simulink model "rover_control"  (R2019b)
settings: Solver=ode3  StartTime=0.0  StopTime=inf  RelTol=1e-3  EnableMultiTasking=on
undefined symbols (not defined in the file or in its folder): Discrete, Time
libraries: embdlinuxlib x13, simulink x3, ctrlSharedLib x2, raspberrypilib x2, sensehatlib x1
(part 1 of 2)
settings Model: DataDictionary=common.sldd  FPTRunName=Active  SimulationMode=external  ExtModeBatchMode=on  ExtModeTrigDuration=100  ExtModeArchiveFileName=rover  ExtModeArchiveDirName=C:\Users\nmb\Desktop\MarsRover\log  ExtModeAddSuffixToVar=on  Creator=nmb  LastModifiedBy=nmb
settings SolverCC: PositivePriorityOrder=on
settings DataIOCC: LimitDataPoints=on  SaveFormat=Array
settings OptimizationCC: ExpressionDepthLimit=2147483647  LifeSpan=Inf  MaxStackSize=64
settings DebuggingCC: UnderspecifiedInitializationDetection=Classic  MergeDetectMultiDrivingBlocksExec=none  FcnCallInpInsideContextMsg=warning  AllowSymbolicDim=off  StateNameClashWarn=warning  SFUnexpectedBacktrackingDiag=warning  SFNoUnconditionalDefaultTransitionDiag=warning  SFExecutionAtInitializationDiag=none  ArithmeticOperatorsInVariantConditions=warning
settings HardwareCC: ProdBitPerPointer=32  ProdBitPerSizeT=32  ProdBitPerPtrDiffT=32  ProdLargestAtomicInteger=Long  ProdLargestAtomicFloat=Double  ProdWordSize=32  ProdHWDeviceType=ARM Compatible->ARM Cortex  UseEmbeddedCoderFeatures=off
settings ModelReferenceCC: PropagateSignalLabelsOutOfModel=off
settings SFSimCC: SimUseLocalCustomCode=off  CustomCodeUndefinedFunction=UseInterfaceOnly
settings RTWCC: SystemTargetFile=ert.tlc  HardwareBoard=Raspberry Pi  TemplateMakefile=ert_default_tmf  GenerateReport=on  RTWVerbose=off  RTWUseLocalCustomCode=off  Toolchain=GNU GCC Raspberry Pi  BuildConfiguration=Faster Runs  LaunchReport=on
settings CodeAppCC: ForceParamTrailComments=on  OperatorAnnotations=on  StateflowObjectComments=on  MATLABSourceComments=on
settings ERTTargetCC: MultiwordLength=2048  ERTCustomFileBanners=off  SupportContinuousTime=on  SupportNonInlinedSFcns=on  RemoveResetFunc=off  SupportVariableSizeSignals=on  ModelStepFunctionPrototypeControlCompliant=off  ExtMode=on  ExtModeMexArgs='192.168.35.184' 0 17725  ERTSrcFileBannerTemplate=codertarget_code_template.cgt  ERTHdrFileBannerTemplate=codertarget_code_template.cgt  ERTDataSrcFileTemplate=codertarget_code_template.cgt  ERTDataHdrFileTemplate=codertarget_code_template.cgt
settings ConfigComp: CovMetricSettings=dw  CovHtmlReporting=on  CovSaveCumulativeToWorkspaceVar=on  CovSaveSingleToWorkspaceVar=on  CovExternalEMLEnable=off  CovSFcnEnable=off

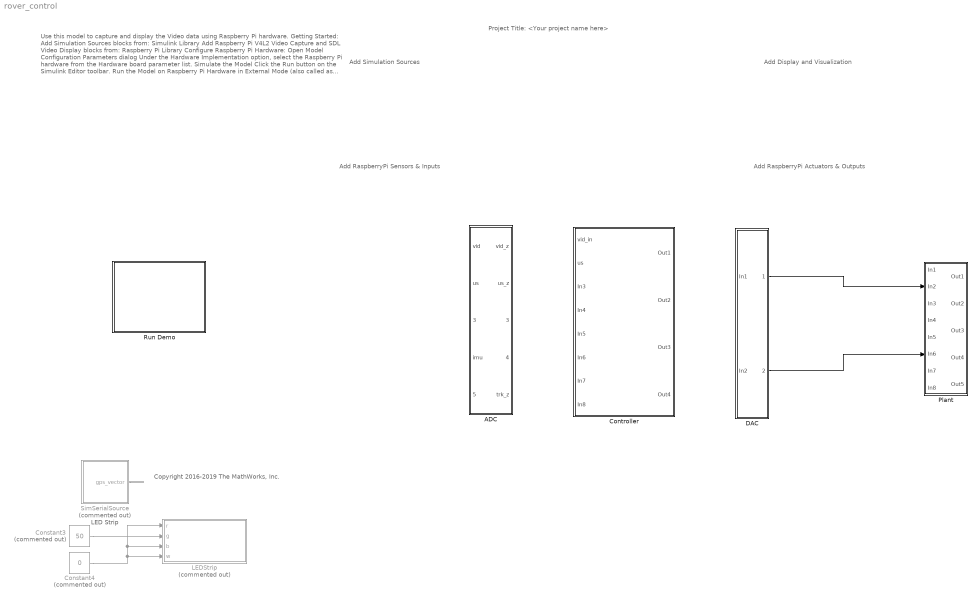
== system rover_control ==
  note: LED Strip
  note: Use this model to capture and display the Video data using Raspberry Pi hardware.
      |
      | Getting Started:
      |
      | Add Simulation Sources blocks from:
      | Simulink Library
      | Add Raspberry Pi V4L2 Video Capture and SDL Video Display blocks from:
      | Raspberry Pi Library
      |
      | Configure Raspberry Pi Hardware:
      |
      | Open Model Configuration Parameters dialog
      | Under the Hardware Implementation option, select the Raspberry Pi hardware from the Hardware board parameter list.
      |
      | Simulate the Model
      |
      | Click the Run button on the Simulink Editor toolbar.
      |
      | Run the Model on Raspberry Pi Hardware in External Mode (also called as Monitor & Tune)
      |
      | In the Hardware tab, click Monitor & Tune
      |
      | External mode will stop when the number of seconds specified in the Simulation stop time parameter elapses.
      |
      | Learn More
      |
      | V4L2 Video Capture
      |
      | SDL Video Display
  note: Add RaspberryPi Sensors & Inputs
  note: Add Display and Visualization
  note: Project Title: <Your project name here>
  note: Add RaspberryPi Actuators & Outputs
  note: Add Simulation Sources
  note: Copyright 2016-2019 The MathWorks, Inc.
  ADC : Subsystem
  Constant3 : Constant  Commented=on  Value=50  OutDataTypeStr=Inherit: Inherit via back propagation
  Constant4 : Constant  Commented=on  Value=0  OutDataTypeStr=Inherit: Inherit via back propagation
  Controller : Subsystem
  DAC : Subsystem
  LEDStrip : Subsystem  Commented=on  DialogController=linuxDDGCreate  InitFcn=|  mask(Ultrasonic Read){board=Model B+, gpio=12, internalResistor=Off, sampleTime=1, direction=Input, blockPlatform=Raspberry Pi}
      | realtime.internal.validateLinuxBlock(get_param(gcbh,'blockPlatform'), gcbh);
      | realtime.internal.gpioCheckParameters(gcs,gcb);
      | realtime.internal.validateGPIO(gcb);
      mask prompts: gpio "GPIO number:"; internalResistor "Internal resistor:"; sampleTime "Sample time:"; blockPlatform "Block platform:"
      mask help: Reads the logical value of a specified GPIO pin configured as input. Select the GPIO input number. Select the internal resistor. Use only one block per GPIO.
      mask init:
      | h = realtime.internal.BoardInfo(blockPlatform);
      | gpioPinName = h.getGPIOPrimaryFunction(board, gpio);
      | gpioPinName = uint8([gpioPinName, 0]); % Add C string termination character
      | 
      | switch (internalResistor)
      |     case {'Off'}
      |         resistor = 1;
      |     case {'Pull-up'}
      |         resistor = 2;
      |     case {'Pull-down'}
      |         resistor = 3;
      |     otherwise
      |         resistor = 255; %N/A
      | end
      | realtime.internal.linuxGpioRead('MaskInitialization');
      mask Help: eval('realtime.helpView(get_param(gcb, ''blockPlatform''), [realtime.internal.getHelpLinkPrefix(gcb) ''libgpioread''])');
      mask TypeOptions direction: Input | Output
      mask Display:
      | text(0.5, 0.15, 'GPIO 12', 'horizontalAlignment', 'center');
      | image(imread('digitalio.png'),[0.32 0.25 0.35 0.55]);
      | color('blue');
      | text(0.90, 0.90, 'RASPBERRYPI', 'horizontalAlignment', 'right');
      | color('black');
  Plant : Subsystem
  Run Demo : Subsystem  Description=Controls host-side RTDX processing.
      mask Display: pic=imread('raspberrypiMonitorAndTune.png');image(pic);
  SimSerialSource : Subsystem  Commented=on
  wires:
  Constant3/1 -> LEDStrip/2(g)
  Constant4/1 -> LEDStrip/1(r), LEDStrip/3(b), LEDStrip/4(w)
  SimSerialSource/1(gps_vector) -> ?
  ? -> ADC/1(vid)
  ? -> ADC/2(us)
  ? -> ADC/3(gps_ser)
  ? -> ADC/4(imu)
  ? -> ADC/5(tracking)
  DAC/1(Out1) -> Plant/2(In2)
  DAC/2(Out2) -> Plant/6(In6)

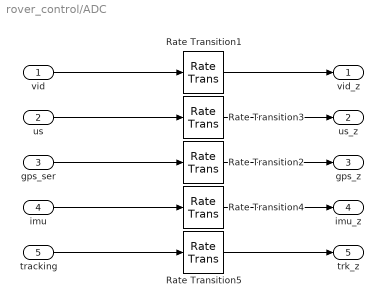
== system rover_control/ADC ==
  vid : Inport
  us : Inport  Port=2
  gps_ser : Inport  Port=3
  imu : Inport  Port=4
  tracking : Inport  Port=5
  Rate Transition{1..5} (5 alike) : RateTransition
  vid_z : Outport
  us_z : Outport  Port=2
  gps_z : Outport  Port=3
  imu_z : Outport  Port=4
  trk_z : Outport  Port=5
  wires:
  Rate Transition3/1 -> us_z/1
  us/1 -> Rate Transition3/1
  vid/1 -> Rate Transition1/1
  Rate Transition1/1 -> vid_z/1
  Rate Transition2/1 -> gps_z/1
  Rate Transition4/1 -> imu_z/1
  gps_ser/1 -> Rate Transition2/1
  imu/1 -> Rate Transition4/1
  tracking/1 -> Rate Transition5/1
  Rate Transition5/1 -> trk_z/1

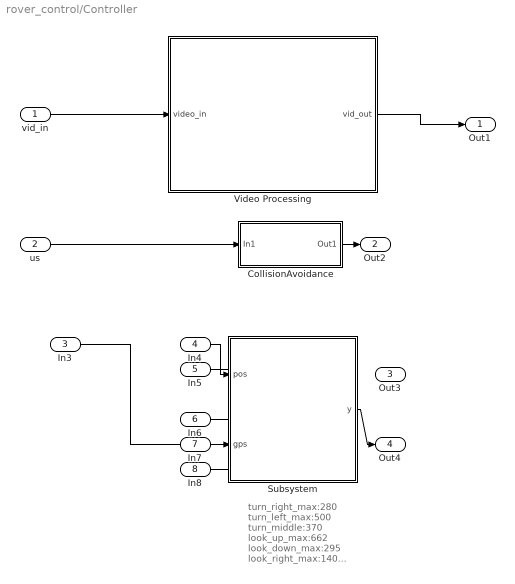
== system rover_control/Controller ==
  note: turn_right_max:280
      | turn_left_max:500
      | turn_middle:370
      | look_up_max:662
      | look_down_max:295
      | look_right_max:140
      | look_left_max:476
  vid_in : Inport
  us : Inport  Port=2
  In3 : Inport  Port=3
  In4 : Inport  Port=4
  In5 : Inport  Port=5
  In6 : Inport  Port=6
  In7 : Inport  Port=7
  In8 : Inport  Port=8
  CollisionAvoidance : Subsystem
  Subsystem : Subsystem
  Video Processing : Subsystem
  Out1 : Outport
  Out2 : Outport  Port=2
  Out3 : Outport  Port=3
  Out4 : Outport  Port=4
  wires:
  In8/1 -> ?
  ? -> Out3/1
  In5/1 -> ?
  vid_in/1 -> Video Processing/1(video_in)
  In7/1 -> ?
  CollisionAvoidance/1(Out1) -> Out2/1
  us/1 -> CollisionAvoidance/1(In1)
  In4/1 -> Subsystem/1(pos)
  In6/1 -> ?
  Subsystem/1(y) -> Out4/1
  In3/1 -> Subsystem/2(gps)
  Video Processing/1(vid_out) -> Out1/1

== system rover_control/DAC ==
  In1 : Inport
  In2 : Inport  Port=2
  Rate Transition : RateTransition  OutPortSampleTime=0.5
  Rate Transition1 : RateTransition  OutPortSampleTime=0.5
  Out1 : Outport
  Out2 : Outport  Port=2
  wires:
  In2/1 -> Rate Transition1/1
  In1/1 -> Rate Transition/1
  Rate Transition1/1 -> Out2/1
  Rate Transition/1 -> Out1/1

== system rover_control/LEDStrip ==
  r : Inport
  g : Inport  Port=2
  b : Inport  Port=3
  w : Inport  Port=4
  MATLAB System : MATLABSystem  System=WS2812  OutputPin=gpio  SampleTime=sampleTime
      mask Type: WS2812
      mask Display: disp('WS2812');
  wires:
  r/1 -> MATLAB System/1
  g/1 -> MATLAB System/2
  b/1 -> MATLAB System/3
  w/1 -> MATLAB System/4

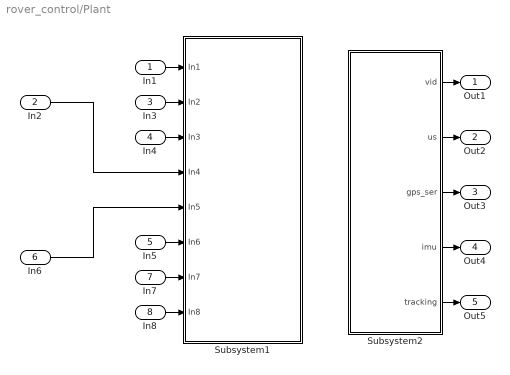
== system rover_control/Plant ==
  In1 : Inport
  In2 : Inport  Port=2
  In3 : Inport  Port=3
  In4 : Inport  Port=4
  In5 : Inport  Port=5
  In6 : Inport  Port=6
  In7 : Inport  Port=7
  In8 : Inport  Port=8
  Subsystem1 : Subsystem  VariantControlMode=Label  Variant=on  VariantControl=Variant1  LabelModeActiveChoice=Variant1
  Subsystem2 : Subsystem  VariantControlMode=Label  Variant=on  VariantControl=Variant1  LabelModeActiveChoice=Variant1
  Out1 : Outport
  Out2 : Outport  Port=2
  Out3 : Outport  Port=3
  Out4 : Outport  Port=4
  Out5 : Outport  Port=5
  wires:
  In3/1 -> Subsystem1/2(In2)
  Subsystem2/2(us) -> Out2/1
  Subsystem2/3(gps_ser) -> Out3/1
  Subsystem2/4(imu) -> Out4/1
  Subsystem2/1(vid) -> Out1/1
  In8/1 -> Subsystem1/8(In8)
  Subsystem2/5(tracking) -> Out5/1
  In2/1 -> Subsystem1/4(In4)
  In7/1 -> Subsystem1/7(In7)
  In6/1 -> Subsystem1/5(In5)
  In1/1 -> Subsystem1/1(In1)
  In4/1 -> Subsystem1/3(In3)
  In5/1 -> Subsystem1/6(In6)

== system rover_control/Run Demo ==

== system rover_control/SimSerialSource ==
  Zero : Constant  Value=uint8(zeros(1,164))  OutDataTypeStr=Inherit: Inherit via back propagation
  gps_vector : Outport
  wires:
  Zero/1 -> gps_vector/1  "gps_vector"

== system rover_control/Controller/CollisionAvoidance ==
  In1 : Inport  SampleTime=0.06
  Chart : Stateflow chart  BlockKeywords=__PRM__SERIALIZED__DATA__:Stateflow Chart,Stateflow Diagram  TreatAsAtomicUnit=on
  Ground : Ground
  Kalman Filter : ctrlSharedLib/Kalman Filter  TimeDomain=Discrete-Time  UseCurrentEstimator=on  ModelSource=Individual A, B, C, D matrices  ModelSourceVariable=ss(0.95,1,1,0,1)  A=[1 0.06; 0 1]  B=1  C=[1 1]  D=0  NumberOfStates=1  NumberOfInputs=1  NumberOfOutputs=1  InitialEstimateSource=Dialog  X0=0  P0=10  UseK=off  UseGH=off  NumberOfProcessNoiseInputs=1  G=[0.1/2 0;1 0]  TimeInvariantG=on  H=0  TimeInvariantH=on  Q=0.05  TimeInvariantQ=on  R=50  TimeInvariantR=on  N=0  TimeInvariantN=on  AddInputPort=off  AddEnablePort=off  OutputEstimatedY=off  OutputP=off  Ts=0.06
      settings: SourceProductBaseCode=CT
  Scope : Scope  NumInputPorts=2
  Out1 : Outport
  wires:
  Kalman Filter/1 -> Scope/2, Chart/1(data)
  Ground/1 -> Out1/1
  In1/1 -> Scope/1, Kalman Filter/1

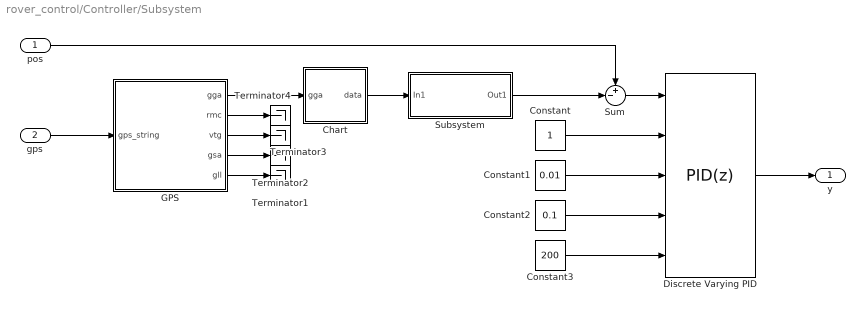
== system rover_control/Controller/Subsystem ==
  pos : Inport
  gps : Inport  Port=2
  Chart : Stateflow chart  BlockKeywords=__PRM__SERIALIZED__DATA__:Stateflow Chart,Stateflow Diagram  TreatAsAtomicUnit=on
  Constant : Constant
  Constant1 : Constant  Value=0.01
  Constant2 : Constant  Value=0.1
  Constant3 : Constant  Value=200
  Discrete Varying PID : simulink/Continuous/PID Controller  Controller=PID  Form=Parallel  TimeDomain=Discrete-time  SampleTime=-1  IntegratorMethod=Forward Euler  FilterMethod=Forward Euler  ControllerParametersSource=external  P=1  I=1  D=0  UseFilter=on  N=100  TunerSelectOption=Transfer Function Based (PID Tuner App)  InitialConditionSource=internal  InitialConditionForIntegrator=0  InitialConditionForFilter=0  DifferentiatorICPrevScaledInput=0  ExternalReset=none  TrackingMode=off  Kt=1  LimitOutput=off  UpperSaturationLimit=inf  LowerSaturationLimit=-inf  LinearizeAsGain=on  AntiWindupMode=none  Kb=1  POutMin=[]  POutMax=[]  IOutMin=[]  IOutMax=[]  DOutMin=[]  DOutMax=[]  NOutMin=[]  NOutMax=[]  SumOutMin=[]  SumOutMax=[]  SaturationOutMin=[]  SaturationOutMax=[]  PParamMin=[]  PParamMax=[]  IParamMin=[]  IParamMax=[]  DParamMin=[]  DParamMax=[]  NParamMin=[]  NParamMax=[]  KbParamMin=[]  KbParamMax=[]  KtParamMin=[]  KtParamMax=[]  KbOutMin=[]  KbOutMax=[]  KtOutMin=[]  KtOutMax=[]  IntegratorOutMin=[]  IntegratorOutMax=[]  FilterOutMin=[]  FilterOutMax=[]  SumI1OutMin=[]  SumI1OutMax=[]  SumI2OutMin=[]  SumI2OutMax=[]  SumI3OutMin=[]  SumI3OutMax=[]  SumI4OutMin=[]  SumI4OutMax=[]  SumDOutMin=[]  SumDOutMax=[]  DifferentiatorOutMin=[]  DifferentiatorOutMax=[]  FilterDiffOutCoefMin=[]  FilterDiffOutCoefMax=[]  ReciprocalOutMin=[]  ReciprocalOutMax=[]  SumDenOutMin=[]  SumDenOutMax=[]  SumNumOutMin=[]  SumNumOutMax=[]  DivideOutMin=[]  DivideOutMax=[]  IntegratorContinuousStateAttributes=''  IntegratorStateMustResolveToSignalObject=off  IntegratorRTWStateStorageClass=Auto  FilterContinuousStateAttributes=''  FilterStateMustResolveToSignalObject=off  FilterRTWStateStorageClass=Auto  ParallelPVariant=ExternalParameters  IdealPVariant=Disabled  IVariant=ExternalParameters  DVariant=ExternalParameters  IntegratorVariant=Discrete  SatVariant=Disabled  AWVariant=Passthrough  PCopyVariant=Disabled  TRVariant=Disabled  FdbkBlocksVariant=Forward  IdealPFdbkVariant=Disabled  SatFdbkVariant=Disabled  DerivativeFilterVariant=ForwardEulerFilter  NVariant=ExternalParameters  NCopyVariant=Disabled  FilterICVariant=InternalICsFilter  IntegratorICVariant=InternalICs  ExternalResetVariant=Disabled  TRSumVariant=Passthrough  SumFdbkVariant=Disabled  SumVariant=Sum_PID
  GPS : Subsystem
  Subsystem : Subsystem
  Sum : Sum  Inputs=+-|
  Terminator{1..4} (4 alike) : Terminator
  y : Outport
  wires:
  GPS/5(gll) -> Terminator1/1
  pos/1 -> Sum/1
  GPS/3(vtg) -> Terminator3/1
  GPS/4(gsa) -> Terminator2/1
  Constant3/1 -> Discrete Varying PID/5
  Constant/1 -> Discrete Varying PID/2
  Constant2/1 -> Discrete Varying PID/4
  GPS/2(rmc) -> Terminator4/1
  GPS/1(gga) -> Chart/1(gga)
  Discrete Varying PID/1 -> y/1
  Constant1/1 -> Discrete Varying PID/3
  gps/1 -> GPS/1(gps_string)
  Chart/1(data) -> Subsystem/1(In1)
  Sum/1 -> Discrete Varying PID/1
  Subsystem/1(Out1) -> Sum/2

== system rover_control/Controller/Video Processing ==
  video_in : Inport
  vid_out : Outport
  wires:
  video_in/1 -> vid_out/1

== system rover_control/Plant/Subsystem1 ==
  In1 : Inport
  In2 : Inport  Port=2
  In3 : Inport  Port=3
  In4 : Inport  Port=4
  In5 : Inport  Port=5
  In6 : Inport  Port=6
  In7 : Inport  Port=7
  In8 : Inport  Port=8
  Subsystem1 : Subsystem  VariantControl=Variant1

== system rover_control/Plant/Subsystem2 ==
  RPiSystem : Subsystem  VariantControl=Variant1
  vid : Outport
  us : Outport  Port=2
  gps_ser : Outport  Port=3
  imu : Outport  Port=4
  tracking : Outport  Port=5

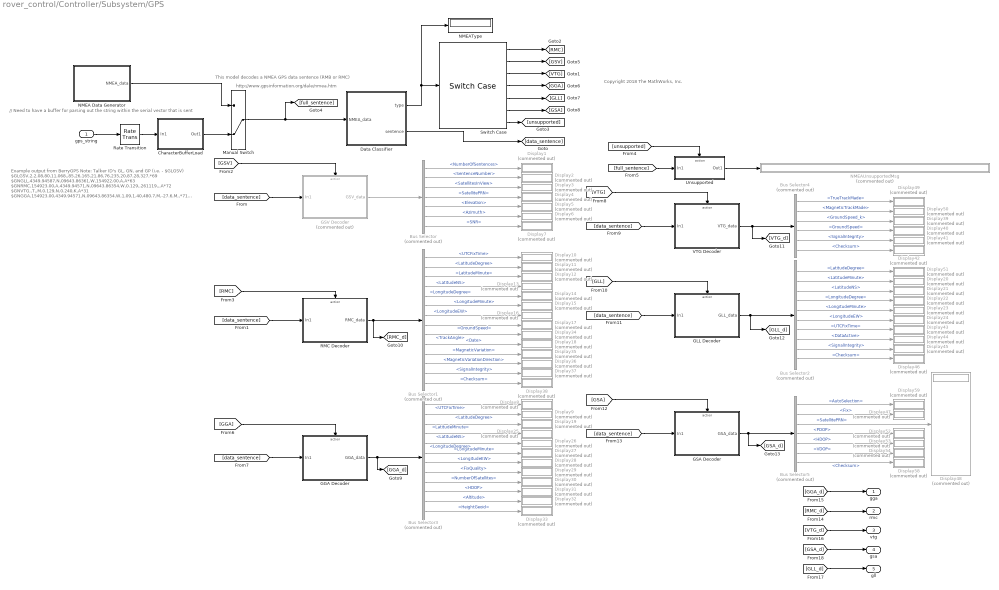
== system rover_control/Controller/Subsystem/GPS ==
  note: // Need to have a buffer for parsing out the string within the serial vector that is sent
  note: Example output from BerryGPS
      | Note: Talker ID's GL, GN, and GP (i.e. - $GLGSV)
      |
      | $GLGSV,2,2,08,80,11,068,,85,26,165,21,86,76,235,20,87,28,327,*69
      | $GNGLL,4349.94587,N,09643.86361,W,154922.00,A,A*63
      | $GNRMC,154923.00,A,4349.94571,N,09643.86354,W,0.129,,261119,,,A*72
      | $GNVTG,,T,,M,0.129,N,0.240,K,A*31
      | $GNGGA,154923.00,4349.94571,N,09643.86354,W,1,09,1.40,480.7,M,-27.6,M,,*71
      | $GNGSA,A,3,32,21,20,29,13,15,,,,,,,1.95,1.40,1.35*1E
      | $GNGSA,A,3,85,71,70,,,,,,,,,,1.95,1.40,1.35*1F
      | $GPGSV,3,1,10,08,05,331,,10,41,276,19,13,19,044,11,15,49,058,26*73
      | $GPGSV,3,2,10,20,68,302,16,21,84,181,17,24,25,126,15,27,28,306,*78
      | $GPGSV,3,3,10,29,09,180,12,32,10,214,27*72
      | $GLGSV,2,1,08,70,31,044,15,71,73,335,10,72,36,249,,79,08,018,*69
      | $GLGSV,2,2,08,80,11,068,,85,26,165,20,86,76,235,20,87,28,327,*68
      | $GNGLL,4349.94571,N,09643.86354,W,154923.00,A,A*6D
      | $GNRMC,154924.00,A,4349.94580,N,09643.86402,W,0.280,,261119,,,A*7F
      | $GNVTG,,T,,M,0.280,N,0.518,K,A*3B
      | $GNGGA,154924.00,4349.94580,N,09643.86402,W,1,09,1.40,481.1,M,-27.6,M,,*7B
      | $GNGSA,A,3,32,21,20,29,13,15,,,,,,,1.95,1.40,1.35*1E
      | $GNGSA,A,3,85,71,70,,,,,,,,,,1.95,1.40,1.35*1F
      | $GPGSV,3,1,10,08,05,331,,10,41,276,19,13,19,044,11,15,49,058,27*72
      | $GPGSV,3,2,10,20,68,303,17,21,84,181,18,24,25,126,15,27,28,306,*77
      | $GPGSV,3,3,10,29,09,180,10,32,10,214,27*70
      | $GLGSV,2,1,08,70,31,044,11,71,73,335,10,72,36,249,,79,08,018,*6D
      | $GLGSV,2,2,08,80,11,068,,85,26,165,21,86,76,235,20,87,28,327,*69
      | $GNGLL,4349.94580,N,09643.86402,W,154924.00,A,A*60
      | $GNRMC,154925.00,A,4349.94623,N,09643.86468,W,0.724,,261119,,,A*73
      | $GNVTG,,T,,M,0.724,N,1.340,K,A*3A
      | $GNGGA,154925.00,4349.94623,N,09643.86468,W,1,09,1.40,480.9,M,-27.6,M,,*75
      | $GNGSA,A,3,32,21,20,29,13,15,,,,,,,1.95,1.40,1.35*1E
      | $GNGSA,A,3,85,71,70,,,,,,,,,,1.95,1.40,1.35*1F
      | $GPGSV,3,1,10,08,05,331,,10,41,276,19,13,19,044,12,15,49,058,27*71
      | $GPGSV,3,2,10,20,68,303,16,21,84,179,18,24,25,126,13,27,28,306,*77
      | $GPGSV,3,3,10,29,09,180,13,32,10,214,27*73
      | $GLGSV,2,1,08,70,31,044,11,71,73,335,07,72,36,249,,79,08,018,*6B
      | $GLGSV,2,2,08,80,11,068,,85,26,165,21,86,76,235,20,87,28,327,*69
      | $GNGLL,4349.94623,N,09643.86468,W,154925.00,A,A*67
  note: Copyright 2018 The MathWorks, Inc.
  note: This model decodes a NMEA GPS data sentence (RMB or RMC)
  note: http://www.gpsinformation.org/dale/nmea.htm
  gps_string : Inport
  Bus Selector : BusSelector  Commented=on  OutputSignals=NumberOfSentences,SentenceNumber,SatellitesInView,SatellitePRN,Elevation,Azimuth,SNR
  Bus Selector1 : BusSelector  Commented=on  OutputSignals=UTCFixTime,LatitudeDegree,LatitudeMinute,LatitudeNS,LongitudeDegree,LongitudeMinute,LongitudeEW,GroundSpeed,TrackAngle,Date,MagneticVariation,MagneticVariationDirection,SignalIntegrity,Checksum
  Bus Selector2 : BusSelector  Commented=on  OutputSignals=LatitudeDegree,LatitudeMinute,LatitudeNS,LongitudeDegree,LongitudeMinute,LongitudeEW,UTCFixTime,DataActive,SignalIntegrity,Checksum
  Bus Selector3 : BusSelector  Commented=on  OutputSignals=UTCFixTime,LatitudeDegree,LatitudeMinute,LatitudeNS,LongitudeDegree,LongitudeMinute,LongitudeEW,FixQuality,NumberOfSatellites,HDOP,Altitude,HeightGeoid
  Bus Selector4 : BusSelector  Commented=on  OutputSignals=TrueTrackMade,MagneticTrackMade,GroundSpeed_k,GroundSpeed,SignalIntegrity,Checksum
  Bus Selector5 : BusSelector  Commented=on  OutputSignals=AutoSelection,Fix,SatellitePRN,PDOP,HDOP,VDOP,Checksum
  CharacterBufferLoad : Subsystem
  Data Classifier : Subsystem  TreatAsAtomicUnit=on
  Display{1..54,58..59} (56 alike) : Display  Commented=on
  GGA Decoder : Subsystem
  GLL Decoder : Subsystem
  GSA Decoder : Subsystem
  GSV Decoder : Subsystem  Commented=on
  Manual Switch : ManualSwitch  CurrentSetting=0
  NMEA Data Generator : Subsystem
  NMEAType : Display
  NMEAUnsupportedMsg : Display  Commented=on
  RMC Decoder : Subsystem
  Rate Transition : RateTransition  OutPortSampleTime=0.05
  Switch Case : SwitchCase  CaseConditions={NMEASentence.RMC, NMEASentence.GSV, NMEASentence.VTG, NMEASentence.GGA, NMEASentence.GLL, NMEASentence.GSA}
  Unsupported : Subsystem
  VTG Decoder : Subsystem
  gga : Outport
  rmc : Outport  Port=2
  vtg : Outport  Port=3
  gsa : Outport  Port=4
  gll : Outport  Port=5
  wires:
  gps_string/1 -> Rate Transition/1
  Bus Selector/2 -> Display2/1  "<SentenceNumber>"
  Bus Selector1/2 -> Display11/1  "<LatitudeDegree>"
  Bus Selector/5 -> Display5/1  "<Elevation>"
  Bus Selector1/3 -> Display12/1  "<LatitudeMinute>"
  Bus Selector/3 -> Display3/1  "<SatellitesInView>"
  Bus Selector/4 -> Display4/1  "<SatellitePRN>"
  Bus Selector/6 -> Display6/1  "<Azimuth>"
  Bus Selector1/7 -> Display16/1  "<LongitudeEW>"
  Bus Selector1/10 -> Display18/1  "<Date>"
  Bus Selector1/6 -> Display15/1  "<LongitudeMinute>"
  Bus Selector1/1 -> Display10/1  "<UTCFixTime>"
  GSV Decoder/1(GSV_data) -> Bus Selector/1
  Data Classifier/1(type) -> NMEAType/1, Switch Case/1
  Unsupported/1(Out1) -> NMEAUnsupportedMsg/1
  [full_sentence] -> Unsupported/1(In1)
  [GSV] -> GSV Decoder/Action
  Data Classifier/2(sentence) -> [data_sentence]
  Bus Selector/1 -> Display1/1  "<NumberOfSentences>"
  Manual Switch/1 -> [full_sentence], Data Classifier/1(NMEA_data)
  [RMC] -> RMC Decoder/Action
  Bus Selector1/4 -> Display13/1  "<LatitudeNS>"
  Switch Case/1 -> [RMC]
  [data_sentence] -> RMC Decoder/1(In1)
  Switch Case/2 -> [GSV]
  [unsupported] -> Unsupported/Action
  RMC Decoder/1(RMC_data) -> [RMC_d], Bus Selector1/1
  Bus Selector1/5 -> Display14/1  "<LongitudeDegree>"
  Bus Selector1/8 -> Display17/1  "<GroundSpeed>"
  Bus Selector/7 -> Display7/1  "<SNR>"
  Switch Case/7 -> [unsupported]
  [data_sentence] -> GSV Decoder/1(In1)
  Switch Case/3 -> [VTG]
  [GGA] -> GGA Decoder/Action
  [data_sentence] -> GGA Decoder/1(In1)
  GGA Decoder/1(GGA_data) -> [GGA_d], Bus Selector3/1
  Bus Selector3/1 -> Display8/1  "<UTCFixTime>"
  Bus Selector3/2 -> Display9/1  "<LatitudeDegree>"
  Bus Selector3/3 -> Display19/1  "<LatitudeMinute>"
  Bus Selector3/4 -> Display25/1  "<LatitudeNS>"
  Switch Case/4 -> [GGA]
  Switch Case/5 -> [GLL]
  Switch Case/6 -> [GSA]
  Rate Transition/1 -> CharacterBufferLoad/1(In1)
  CharacterBufferLoad/1(Out1) -> Manual Switch/2
  NMEA Data Generator/1(NMEA_data) -> Manual Switch/1
  Bus Selector3/6 -> Display27/1  "<LongitudeMinute>"
  Bus Selector3/7 -> Display28/1  "<LongitudeEW>"
  Bus Selector3/8 -> Display29/1  "<FixQuality>"
  Bus Selector3/9 -> Display30/1  "<NumberOfSatellites>"
  Bus Selector3/10 -> Display31/1  "<HDOP>"
  Bus Selector3/11 -> Display32/1  "<Altitude>"
  Bus Selector3/12 -> Display33/1  "<HeightGeoid>"
  Bus Selector3/5 -> Display26/1  "<LongitudeDegree>"
  Bus Selector1/9 -> Display34/1  "<TrackAngle>"
  Bus Selector1/11 -> Display35/1  "<MagneticVariation>"
  Bus Selector1/12 -> Display36/1  "<MagneticVariationDirection>"
  Bus Selector1/13 -> Display37/1  "<SignalIntegrity>"
  Bus Selector1/14 -> Display38/1  "<Checksum>"
  Bus Selector4/5 -> Display41/1  "<SignalIntegrity>"
  Bus Selector4/6 -> Display42/1  "<Checksum>"
  VTG Decoder/1(VTG_data) -> [VTG_d], Bus Selector4/1
  [VTG] -> VTG Decoder/Action
  Bus Selector4/4 -> Display40/1  "<GroundSpeed>"
  Bus Selector4/2 -> Display50/1  "<MagneticTrackMade>"
  Bus Selector4/3 -> Display39/1  "<GroundSpeed_k>"
  [data_sentence] -> VTG Decoder/1(In1)
  Bus Selector4/1 -> Display49/1  "<TrueTrackMade>"
  Bus Selector2/4 -> Display22/1  "<LongitudeDegree>"
  Bus Selector2/10 -> Display46/1  "<Checksum>"
  Bus Selector2/9 -> Display45/1  "<SignalIntegrity>"
  Bus Selector2/8 -> Display44/1  "<DataActive>"
  Bus Selector2/7 -> Display43/1  "<UTCFixTime>"
  Bus Selector2/6 -> Display24/1  "<LongitudeEW>"
  Bus Selector2/5 -> Display23/1  "<LongitudeMinute>"
  Bus Selector2/3 -> Display21/1  "<LatitudeNS>"
  Bus Selector2/2 -> Display20/1  "<LatitudeMinute>"
  Bus Selector2/1 -> Display51/1  "<LatitudeDegree>"
  GLL Decoder/1(GLL_data) -> [GLL_d], Bus Selector2/1
  [data_sentence] -> GLL Decoder/1(In1)
  [GLL] -> GLL Decoder/Action
  [GSA] -> GSA Decoder/Action
  [data_sentence] -> GSA Decoder/1(In1)
  GSA Decoder/1(GSA_data) -> [GSA_d], Bus Selector5/1
  Bus Selector5/1 -> Display59/1  "<AutoSelection>"
  Bus Selector5/2 -> Display47/1  "<Fix>"
  Bus Selector5/3 -> Display48/1  "<SatellitePRN>"
  Bus Selector5/5 -> Display53/1  "<HDOP>"
  Bus Selector5/6 -> Display54/1  "<VDOP>"
  Bus Selector5/7 -> Display58/1  "<Checksum>"
  Bus Selector5/4 -> Display52/1  "<PDOP>"
  [GGA_d] -> gga/1
  [RMC_d] -> rmc/1
  [VTG_d] -> vtg/1
  [GSA_d] -> gsa/1
  [GLL_d] -> gll/1

== system rover_control/Controller/Subsystem/Subsystem ==
  In1 : Inport
  Kalman Filter : ctrlSharedLib/Kalman Filter  TimeDomain=Discrete-Time  UseCurrentEstimator=on  ModelSource=Individual A, B, C, D matrices  ModelSourceVariable=ss(0.95,1,1,0,1)  A=[1 0 0.1 0;0 1 0 0.1;0 0 1 0;0 0 0 1]  B=1  C=[1 0 0 0;0 1 0 0];  D=0  NumberOfStates=1  NumberOfInputs=1  NumberOfOutputs=1  InitialEstimateSource=Dialog  X0=0  P0=10  UseK=off  UseGH=on  NumberOfProcessNoiseInputs=1  G=[0.1/2 0;0 0.1/2; 1 0; 0 1]  TimeInvariantG=on  H=0  TimeInvariantH=on  Q=0.05  TimeInvariantQ=on  R=1  TimeInvariantR=on  N=0  TimeInvariantN=on  AddInputPort=on  AddEnablePort=off  OutputEstimatedY=off  OutputP=off  Ts=-1
      settings: SourceProductBaseCode=CT
  Out1 : Outport
  wires:
  In1/1 -> Out1/1

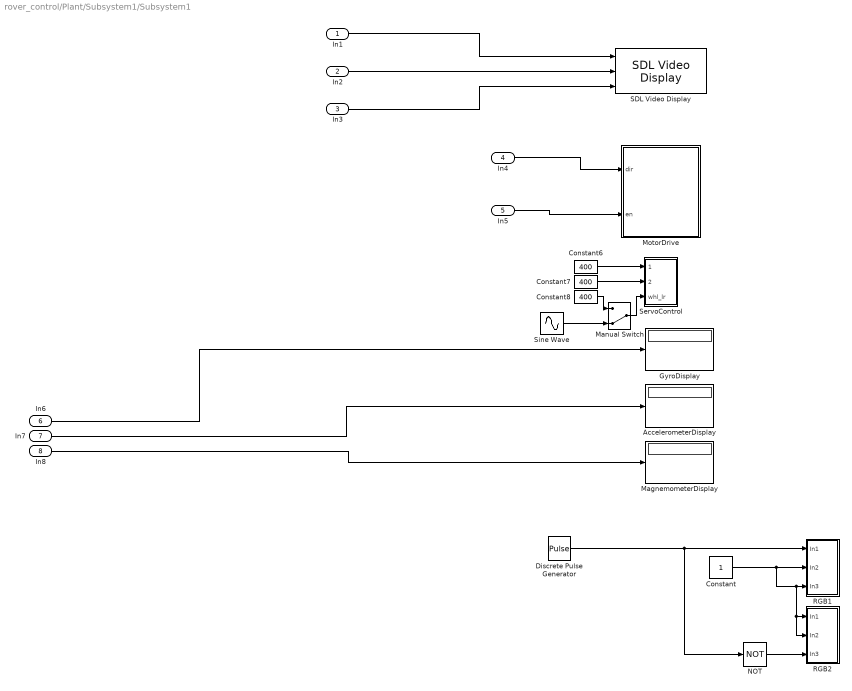
== system rover_control/Plant/Subsystem1/Subsystem1 ==
  In1 : Inport
  In2 : Inport  Port=2
  In3 : Inport  Port=3
  In4 : Inport  Port=4
  In5 : Inport  Port=5
  In6 : Inport  Port=6
  In7 : Inport  Port=7
  In8 : Inport  Port=8
  AccelerometerDisplay : Display
  Constant : Constant
  Constant6 : Constant  Value=400
  Constant7 : Constant  Value=400
  Constant8 : Constant  Value=400
  Discrete Pulse Generator : DiscretePulseGenerator  Period=10  PulseWidth=5  SampleTime=0.25
  GyroDisplay : Display
  MagnemometerDisplay : Display
  Manual Switch : ManualSwitch  CurrentSetting=0
  MotorDrive : Subsystem
  NOT : Logic  Operator=NOT  IconShape=distinctive  AllPortsSameDT=off  OutDataTypeStr=boolean
  RGB1 : Subsystem
  RGB2 : Subsystem
  SDL Video Display : embdlinuxlib/SDL Video Display  pixelFormat=RGB  pixelOrder=Planar  rowMajor=on  blockPlatform=Raspberry Pi
      settings: SourceProductName=Simulink Support Package for Raspberry Pi Hardware  SourceProductBaseCode=RASPPI
  ServoControl : Subsystem  TreatAsAtomicUnit=on  SystemSampleTime=0.05
      settings: RTWSystemCode=Nonreusable function  RTWFcnNameOpts=Use subsystem name
  Sine Wave : Sin  Amplitude=110  Bias=280+110  SampleTime=0.05
  wires:
  Constant6/1 -> ServoControl/1(cam_ud)
  Discrete Pulse Generator/1 -> NOT/1, RGB1/1(In1)
  NOT/1 -> RGB2/3(In3)
  In2/1 -> SDL Video Display/2
  Constant/1 -> RGB2/2(In2), RGB2/1(In1), RGB1/3(In3), RGB1/2(In2)
  Constant8/1 -> Manual Switch/1
  Manual Switch/1 -> ServoControl/3(whl_lr)
  Sine Wave/1 -> Manual Switch/2
  Constant7/1 -> ServoControl/2(cam_lr)
  In6/1 -> GyroDisplay/1
  In3/1 -> SDL Video Display/3
  In7/1 -> AccelerometerDisplay/1
  In4/1 -> MotorDrive/1(dir)
  In1/1 -> SDL Video Display/1
  In5/1 -> MotorDrive/2(en)
  In8/1 -> MagnemometerDisplay/1

== system rover_control/Plant/Subsystem2/RPiSystem ==
  Bus Creator : BusCreator  Inputs=3
  Bus Creator1 : BusCreator  Inputs=3
  LSM9DS1 IMU Sensor : sensehatlib/LSM9DS1 IMU Sensor  blockPlatform=Raspberry Pi  BoardProperty_sh=Pi 3 Model B  ActiveSensors_=Accelerometer, Gyroscope and Magnetometer  AccelerometerOutputDataRate=119 Hz  AccelerometerFullScaleRange=+/- 2g  AccelerometerBandwidth=50 Hz  GyroscopeOutputDataRate=119 Hz  GyroscopeFullScaleRange=245 dps  GyroscopeBandwidthMode=0  GyroscopeHighPassFilterEnabled=off  GyroscopeHighPassFilterMode=0  MagnetometerFullScaleRange=+/- 4 gauss  MagnetometerOutputDataRate=40 Hz  SampleTime=0.1
      settings: SourceProductName=Simulink Support Package for Raspberry Pi Hardware  SourceProductBaseCode=RASPPI
  RPiSerialSource : Subsystem
  Tracking3CH : Subsystem
  UltrasonicSensor : Subsystem  DialogController=linuxDDGCreate  InitFcn=|  mask(Ultrasonic Read){board=Model B+, echo_gpio=8, trigger_gpio=11, internalResistor=Off, sampleTime=0.06, direction=Input, blockPlatform=Raspberry Pi}
      | %realtime.internal.validateLinuxBlock(get_param(gcbh,'blockPlatform'), gcbh);
      | %realtime.internal.gpioCheckParameters(gcs,gcb);
      | %realtime.internal.validateGPIO(gcb);
      mask prompts: echo_gpio "Echo GPIO number:"; trigger_gpio "Trigger GPIO number"; internalResistor "Internal resistor:"; sampleTime "Sample time:"; blockPlatform "Block platform:"
      mask help: Reads the logical value of a specified GPIO pin configured as input. Select the GPIO input number. Select the internal resistor. Use only one block per GPIO.
      mask init:
      | h = realtime.internal.BoardInfo(blockPlatform);
      | echoPinName = h.getGPIOPrimaryFunction(board, echo_gpio);
      | echoPinName = uint8([echoPinName, 0]); % Add C string termination character
      | triggerPinName = h.getGPIOPrimaryFunction(board, trigger_gpio);
      | triggerPinName = uint8([triggerPinName, 0]); % Add C string termination character
      | 
      | switch (internalResistor)
      |     case {'Off'}
      |         resistor = 1;
      |     case {'Pull-up'}
      |         resistor = 2;
      |     case {'Pull-down'}
      |         resistor = 3;
      |     otherwise
      |         resistor = 255; %N/A
      | end
      | %realtime.internal.linuxGpioRead('MaskInitialization');
      mask Help: eval('realtime.helpView(get_param(gcb, ''blockPlatform''), [realtime.internal.getHelpLinkPrefix(gcb) ''libgpioread''])');
      mask TypeOptions direction: Input | Output
      mask Display:
      | text(0.5, 0.15, 'ULTRASONIC', 'horizontalAlignment', 'center');
      | [X, map] = imread('us.png');
      | ultra_im = im2uint8(ind2rgb(X,map));
      | image(ultra_im, [0.32 0.25 0.35 0.55]);
      | %image(imread('digitalio.png'),[0.32 0.25 0.35 0.55]);
      | color('blue');
      | text(0.90, 0.90, 'RASPBERRYPI', 'horizontalAlignment', 'right');
      | color('black');
  V4L2 Video Capture : embdlinuxlib/V4L2 Video Capture  m_devName='/dev/video0'  roi=[0, 0, 640, 480]  imSizeSelection=160x120  imSize=[640, 480]  pixelFormat=RGB  pixelOrder=Planar  sampleTime=1/10  simOutput=Colorbars  blockPlatform=Raspberry Pi
      settings: SourceProductName=Simulink Support Package for Raspberry Pi Hardware  SourceProductBaseCode=RASPPI
  vid : Outport
  us : Outport  Port=2
  gps_ser : Outport  Port=3
  imu : Outport  Port=4
  tracking : Outport  Port=5
  wires:
  UltrasonicSensor/1(Out1) -> us/1
  RPiSerialSource/1(gps_vector) -> gps_ser/1
  V4L2 Video Capture/1 -> Bus Creator/1  "R"
  V4L2 Video Capture/2 -> Bus Creator/2  "G"
  V4L2 Video Capture/3 -> Bus Creator/3  "B"
  Bus Creator/1 -> vid/1
  LSM9DS1 IMU Sensor/1 -> Bus Creator1/1  "gyro"
  LSM9DS1 IMU Sensor/2 -> Bus Creator1/2  "accel"
  LSM9DS1 IMU Sensor/3 -> Bus Creator1/3  "mag"
  Bus Creator1/1 -> imu/1
  Tracking3CH/1(tracking) -> tracking/1

== system rover_control/Controller/Subsystem/GPS/CharacterBufferLoad ==
  In1 : Inport
  NMEASentenceExtract : Subsystem  TreatAsAtomicUnit=on  SystemSampleTime=0.05
  Out1 : Outport
  wires:
  NMEASentenceExtract/1(string) -> Out1/1
  In1/1 -> NMEASentenceExtract/1(serial_vector)

== system rover_control/Controller/Subsystem/GPS/Data Classifier ==
  note: Copyright 2018 The MathWorks, Inc.
  NMEA_data : Inport
  Bias1 : Bias  Bias=1
  Constant : Constant  Value=4  OutDataTypeStr=int32
  Constant1 : Constant  Value=3  OutDataTypeStr=uint8
  String Find : StringFind
  String to Enum : StringToEnum  OutDataTypeStr=Enum: NMEASentence
  Substring : Substring
  Substring1 : Substring  StringFromIdxToEnd=on
  comma : StringConstant  String="\",\""
  type : Outport  VectorParamsAs1DForOutWhenUnconnected=off
  sentence : Outport  Port=2  VectorParamsAs1DForOutWhenUnconnected=off
  wires:
  String Find/1 -> Bias1/1  "first_comma"
  NMEA_data/1 -> String Find/1, Substring/1, Substring1/1
  Constant/1 -> Substring/2
  comma/1 -> String Find/2
  Substring/1 -> String to Enum/1
  Substring1/1 -> sentence/1  "sentence"
  String to Enum/1 -> type/1
  Constant1/1 -> Substring/3
  Bias1/1 -> Substring1/2

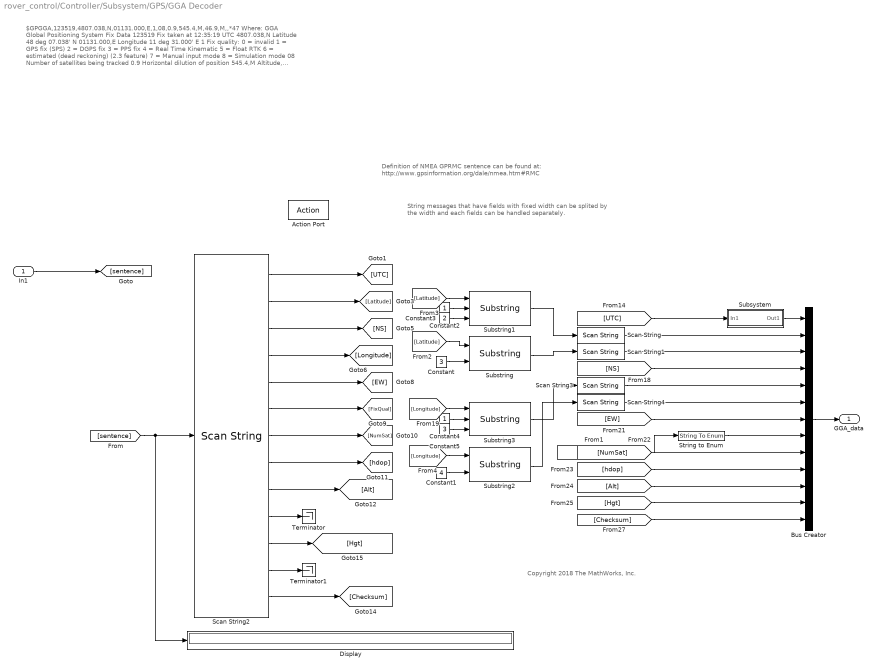
== system rover_control/Controller/Subsystem/GPS/GGA Decoder ==
  note: $GPGGA,123519,4807.038,N,01131.000,E,1,08,0.9,545.4,M,46.9,M,,*47
      |
      | Where:
      | GGA Global Positioning System Fix Data
      | 123519 Fix taken at 12:35:19 UTC
      | 4807.038,N Latitude 48 deg 07.038' N
      | 01131.000,E Longitude 11 deg 31.000' E
      | 1 Fix quality: 0 = invalid
      | 1 = GPS fix (SPS)
      | 2 = DGPS fix
      | 3 = PPS fix
      | 4 = Real Time Kinematic
      | 5 = Float RTK
      | 6 = estimated (dead reckoning) (2.3 feature)
      | 7 = Manual input mode
      | 8 = Simulation mode
      | 08 Number of satellites being tracked
      | 0.9 Horizontal dilution of position
      | 545.4,M Altitude, Meters, above mean sea level
      | 46.9,M Height of geoid (mean sea level) above WGS84
      | ellipsoid
      | (empty field) time in seconds since last DGPS update
      | (empty field) DGPS station ID number
      | *47 the checksum data, always begins with *
  note: Copyright 2018 The MathWorks, Inc.
  note: String messages that have fields with fixed width can be splited
      | by the width and each fields can be handled separately.
  note: Definition of NMEA GPRMC sentence can be found at:
      | http://www.gpsinformation.org/dale/nmea.htm#RMC
  In1 : Inport
  Action Port : ActionPort  ActionPortLabel=case [ GGA ]:
  Bus Creator : BusCreator  Inputs=13  OutDataTypeStr=Bus: NMEA_GPGGA  NonVirtualBus=on
      settings: InheritFromInputs=off
  Constant : Constant  Value=3  OutDataTypeStr=Inherit: Inherit via back propagation
  Constant1 : Constant  Value=4  OutDataTypeStr=Inherit: Inherit via back propagation
  Constant2 : Constant  OutDataTypeStr=Inherit: Inherit via back propagation
  Constant3 : Constant  Value=2  OutDataTypeStr=Inherit: Inherit via back propagation
  Constant4 : Constant  OutDataTypeStr=Inherit: Inherit via back propagation
  Constant5 : Constant  Value=3  OutDataTypeStr=Inherit: Inherit via back propagation
  Display : Display
  Scan String : ScanString  Format="\"%hu\""
  Scan String1 : ScanString  Format="\"%lf\""
  Scan String2 : ScanString  Format="\"%9s,%10s,%1s,%11s,%1s,%1s,%hu,%lf,%lf,%s,%lf,%s,*%s\""
  Scan String3 : ScanString  Format="\"%hu\""
  Scan String4 : ScanString  Format="\"%lf\""
  String to Enum : StringToEnum  OutDataTypeStr=Enum: NMEAFixQuality
  Substring : Substring  StringFromIdxToEnd=on
  Substring1 : Substring
  Substring2 : Substring  StringFromIdxToEnd=on
  Substring3 : Substring
  Subsystem : Subsystem
  Terminator : Terminator
  Terminator1 : Terminator
  GGA_data : Outport  VectorParamsAs1DForOutWhenUnconnected=off
  wires:
  In1/1 -> [sentence]
  Scan String2/1 -> [UTC]
  Scan String2/2 -> [Latitude]
  Scan String2/3 -> [NS]
  Scan String2/4 -> [Longitude]
  Scan String2/5 -> [EW]
  Bus Creator/1 -> GGA_data/1
  [UTC] -> Subsystem/1(In1)
  Scan String/1 -> Bus Creator/2
  [NS] -> Bus Creator/4
  Scan String3/1 -> Bus Creator/5
  [FixQual] -> String to Enum/1
  [Checksum] -> Bus Creator/13
  Scan String1/1 -> Bus Creator/3
  Scan String4/1 -> Bus Creator/6
  [EW] -> Bus Creator/7
  [NumSat] -> Bus Creator/9
  [hdop] -> Bus Creator/10
  [Hgt] -> Bus Creator/12
  Subsystem/1(Out1) -> Bus Creator/1
  [Alt] -> Bus Creator/11
  [sentence] -> Display/1, Scan String2/1
  Scan String2/12 -> Terminator1/1
  String to Enum/1 -> Bus Creator/8
  Scan String2/6 -> [FixQual]
  Scan String2/7 -> [NumSat]
  Scan String2/8 -> [hdop]
  Scan String2/9 -> [Alt]
  Scan String2/10 -> Terminator/1
  Scan String2/11 -> [Hgt]
  Scan String2/13 -> [Checksum]
  [Latitude] -> Substring/1
  Constant/1 -> Substring/2
  Constant3/1 -> Substring1/3
  Constant2/1 -> Substring1/2
  [Latitude] -> Substring1/1
  [Longitude] -> Substring3/1
  Constant4/1 -> Substring3/2
  Constant5/1 -> Substring3/3
  Constant1/1 -> Substring2/2
  [Longitude] -> Substring2/1
  Substring1/1 -> Scan String/1
  Substring/1 -> Scan String1/1
  Substring3/1 -> Scan String3/1
  Substring2/1 -> Scan String4/1

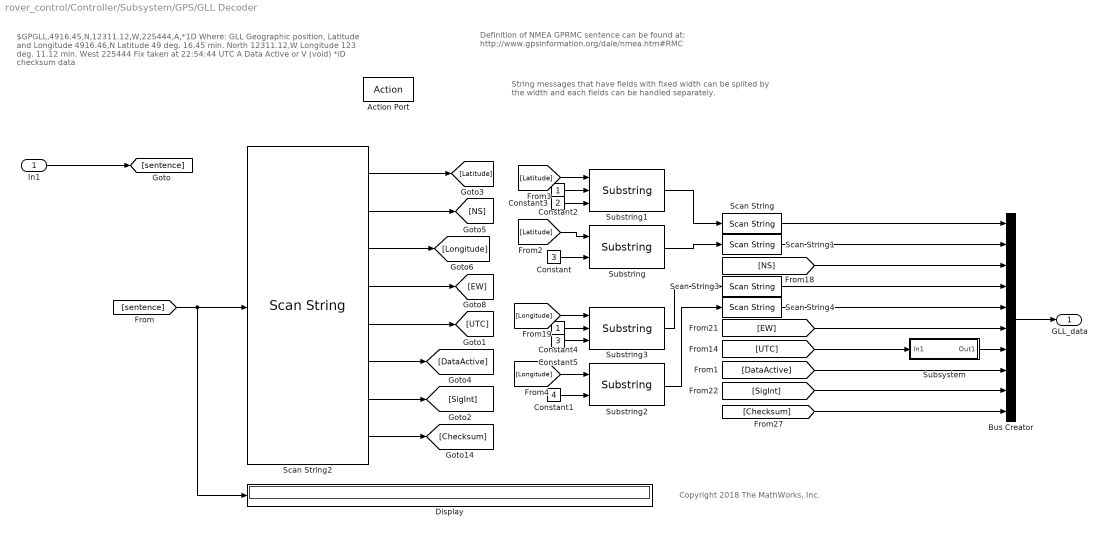
== system rover_control/Controller/Subsystem/GPS/GLL Decoder ==
  note: Definition of NMEA GPRMC sentence can be found at:
      | http://www.gpsinformation.org/dale/nmea.htm#RMC
  note: String messages that have fields with fixed width can be splited
      | by the width and each fields can be handled separately.
  note: Copyright 2018 The MathWorks, Inc.
  note: $GPGLL,4916.45,N,12311.12,W,225444,A,*1D
      |
      | Where:
      | GLL Geographic position, Latitude and Longitude
      | 4916.46,N Latitude 49 deg. 16.45 min. North
      | 12311.12,W Longitude 123 deg. 11.12 min. West
      | 225444 Fix taken at 22:54:44 UTC
      | A Data Active or V (void)
      | *iD checksum data
  In1 : Inport
  Action Port : ActionPort  ActionPortLabel=case [ GLL ]:
  Bus Creator : BusCreator  Inputs=10  OutDataTypeStr=Bus: NMEA_GLL  NonVirtualBus=on
      settings: InheritFromInputs=off
  Constant : Constant  Value=3  OutDataTypeStr=Inherit: Inherit via back propagation
  Constant1 : Constant  Value=4  OutDataTypeStr=Inherit: Inherit via back propagation
  Constant2 : Constant  OutDataTypeStr=Inherit: Inherit via back propagation
  Constant3 : Constant  Value=2  OutDataTypeStr=Inherit: Inherit via back propagation
  Constant4 : Constant  OutDataTypeStr=Inherit: Inherit via back propagation
  Constant5 : Constant  Value=3  OutDataTypeStr=Inherit: Inherit via back propagation
  Display : Display
  Scan String : ScanString  Format="\"%hu\""
  Scan String1 : ScanString  Format="\"%lf\""
  Scan String2 : ScanString  Format="\"%10s,%1s,%11s,%1s,%9s,%1s,%1s,*%2s\""
  Scan String3 : ScanString  Format="\"%hu\""
  Scan String4 : ScanString  Format="\"%lf\""
  Substring : Substring  StringFromIdxToEnd=on
  Substring1 : Substring
  Substring2 : Substring  StringFromIdxToEnd=on
  Substring3 : Substring
  Subsystem : Subsystem
  GLL_data : Outport  VectorParamsAs1DForOutWhenUnconnected=off
  wires:
  Substring2/1 -> Scan String4/1
  Substring3/1 -> Scan String3/1
  Substring/1 -> Scan String1/1
  Substring1/1 -> Scan String/1
  [Longitude] -> Substring2/1
  Constant1/1 -> Substring2/2
  Constant5/1 -> Substring3/3
  Constant4/1 -> Substring3/2
  [Longitude] -> Substring3/1
  [Latitude] -> Substring1/1
  Constant2/1 -> Substring1/2
  Constant3/1 -> Substring1/3
  Constant/1 -> Substring/2
  [Latitude] -> Substring/1
  Scan String2/8 -> [Checksum]
  [DataActive] -> Bus Creator/8
  [sentence] -> Display/1, Scan String2/1
  Subsystem/1(Out1) -> Bus Creator/7
  [SigInt] -> Bus Creator/9
  [EW] -> Bus Creator/6
  Scan String4/1 -> Bus Creator/5
  Scan String1/1 -> Bus Creator/2
  [Checksum] -> Bus Creator/10
  Scan String3/1 -> Bus Creator/4
  [NS] -> Bus Creator/3
  Scan String/1 -> Bus Creator/1
  [UTC] -> Subsystem/1(In1)
  Bus Creator/1 -> GLL_data/1
  Scan String2/4 -> [EW]
  Scan String2/3 -> [Longitude]
  Scan String2/2 -> [NS]
  Scan String2/1 -> [Latitude]
  Scan String2/5 -> [UTC]
  In1/1 -> [sentence]
  Scan String2/7 -> [SigInt]
  Scan String2/6 -> [DataActive]

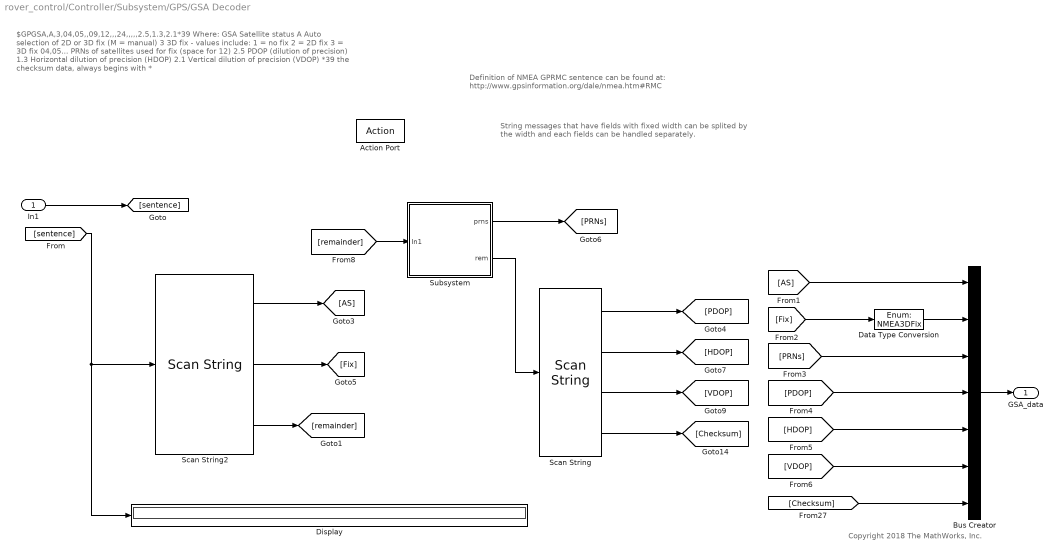
== system rover_control/Controller/Subsystem/GPS/GSA Decoder ==
  note: $GPGSA,A,3,04,05,,09,12,,,24,,,,,2.5,1.3,2.1*39
      |
      | Where:
      | GSA Satellite status
      | A Auto selection of 2D or 3D fix (M = manual)
      | 3 3D fix - values include: 1 = no fix
      | 2 = 2D fix
      | 3 = 3D fix
      | 04,05... PRNs of satellites used for fix (space for 12)
      | 2.5 PDOP (dilution of precision)
      | 1.3 Horizontal dilution of precision (HDOP)
      | 2.1 Vertical dilution of precision (VDOP)
      | *39 the checksum data, always begins with *
  note: Copyright 2018 The MathWorks, Inc.
  note: String messages that have fields with fixed width can be splited
      | by the width and each fields can be handled separately.
  note: Definition of NMEA GPRMC sentence can be found at:
      | http://www.gpsinformation.org/dale/nmea.htm#RMC
  In1 : Inport
  Action Port : ActionPort  ActionPortLabel=case [ GSA ]:
  Bus Creator : BusCreator  Inputs=7  OutDataTypeStr=Bus: NMEA_GSA  NonVirtualBus=on
      settings: InheritFromInputs=off
  Data Type Conversion : DataTypeConversion  OutDataTypeStr=Enum: NMEA3DFix
  Display : Display
  Scan String : ScanString  Format="\"%lf,%lf,%lf,*%2s\""
  Scan String2 : ScanString  Format="\"%1s,%hu,%s\""
  Subsystem : Subsystem
  GSA_data : Outport  VectorParamsAs1DForOutWhenUnconnected=off
  wires:
  In1/1 -> [sentence]
  Scan String2/1 -> [AS]
  Scan String2/2 -> [Fix]
  Bus Creator/1 -> GSA_data/1
  [AS] -> Bus Creator/1
  [PRNs] -> Bus Creator/3
  [PDOP] -> Bus Creator/4
  [Checksum] -> Bus Creator/7
  [Fix] -> Data Type Conversion/1
  [HDOP] -> Bus Creator/5
  [VDOP] -> Bus Creator/6
  [sentence] -> Scan String2/1, Display/1
  Scan String/4 -> [Checksum]
  Scan String/1 -> [PDOP]
  Scan String/2 -> [HDOP]
  Scan String/3 -> [VDOP]
  Data Type Conversion/1 -> Bus Creator/2
  Scan String2/3 -> [remainder]
  [remainder] -> Subsystem/1(In1)
  Subsystem/1(prns) -> [PRNs]
  Subsystem/2(rem) -> Scan String/1

== system rover_control/Controller/Subsystem/GPS/GSV Decoder ==
  note: // todo: there is an error with how this is getting output
  note: $GPGSV,2,1,08,01,40,083,46,02,17,308,41,12,07,344,39,14,22,228,45*75
      |
      | Where:
      | GSV Satellites in view
      | 2 Number of sentences for full data
      | 1 sentence 1 of 2
      | 08 Number of satellites in view
      |
      | 01 Satellite PRN number
      | 40 Elevation, degrees
      | 083 Azimuth, degrees
      | 46 SNR - higher is better
      | for up to 4 satellites per sentence
      | *75 the checksum data, always begins with *
  note: Copyright 2018 The MathWorks, Inc.
  note: Definition of NMEA GPRMB data sentence can be found at:
      | http://www.gpsinformation.org/dale/nmea.htm#RMB
  note: Scan String block is as powerful as sscanf function in C or MATLAB
      | It provides a flexible approach to parse input string message
  In1 : Inport
  Action Port : ActionPort  ActionPortLabel=case [ GSV ]:
  Bus Creator : BusCreator  Inputs=8  OutDataTypeStr=Bus: NMEA_GSV  NonVirtualBus=on
      settings: InheritFromInputs=off
  Data Type Conversion : DataTypeConversion
  Data Type Conversion1 : DataTypeConversion
  Display : Display
  RMB Parser : ScanString  Format="\"%hu,%hu,%hu,%hu,%hu,%hu,%s,*%s\""
  GSV_data : Outport  OutDataTypeStr=Bus: NMEA_GSV  VectorParamsAs1DForOutWhenUnconnected=off
  wires:
  In1/1 -> Display/1, RMB Parser/1
  RMB Parser/1 -> Data Type Conversion/1
  RMB Parser/8 -> Bus Creator/8
  Bus Creator/1 -> GSV_data/1
  RMB Parser/2 -> Data Type Conversion1/1
  RMB Parser/3 -> Bus Creator/3
  RMB Parser/4 -> Bus Creator/4
  RMB Parser/5 -> Bus Creator/5
  RMB Parser/6 -> Bus Creator/6
  RMB Parser/7 -> Bus Creator/7
  Data Type Conversion/1 -> Bus Creator/1
  Data Type Conversion1/1 -> Bus Creator/2

== system rover_control/Controller/Subsystem/GPS/NMEA Data Generator ==
  Multiport Switch : MultiPortSwitch
  Rate Transition1 : RateTransition  OutPortSampleTime=0.05
  Recommended Minimum Navigation Information : StringConstant  String="\"$GPRMB,A,0.66,L,003,004,4917.24,N,12309.57,W,001.3,052.5,000.5,V*20\""
  Recommended Minimum Sentence C : StringConstant  String="\"$GPRMC,123519,A,4807.038,N,01131.000,E,022.4,084.4,230394,003.1,W*6A\""
  Repeating Sequence Stair : simulink/Sources/Repeating Sequence Stair  OutValues=[1 1 1 1 2 2 2 2 3 3 3]  tsamp=1  OutMin=[]  OutMax=[]  OutDataTypeStr=double  OutputDataTypeScalingMode=double  OutDataType=fixdt(0,8)  ConRadixGroup=Best Precision: Vector-wise  OutScaling=2^-12
  Satellite Data : StringConstant  String="\"$GPGSV,2,1,08,01,40,083,46,02,17,308,41,12,07,344,39,14,22,228,45*75\""
  NMEA_data : Outport  VectorParamsAs1DForOutWhenUnconnected=off
  wires:
  Multiport Switch/1 -> NMEA_data/1
  Repeating Sequence Stair/1 -> Rate Transition1/1
  Recommended Minimum Sentence C/1 -> Multiport Switch/3
  Recommended Minimum Navigation Information/1 -> Multiport Switch/2
  Satellite Data/1 -> Multiport Switch/4
  Rate Transition1/1 -> Multiport Switch/1

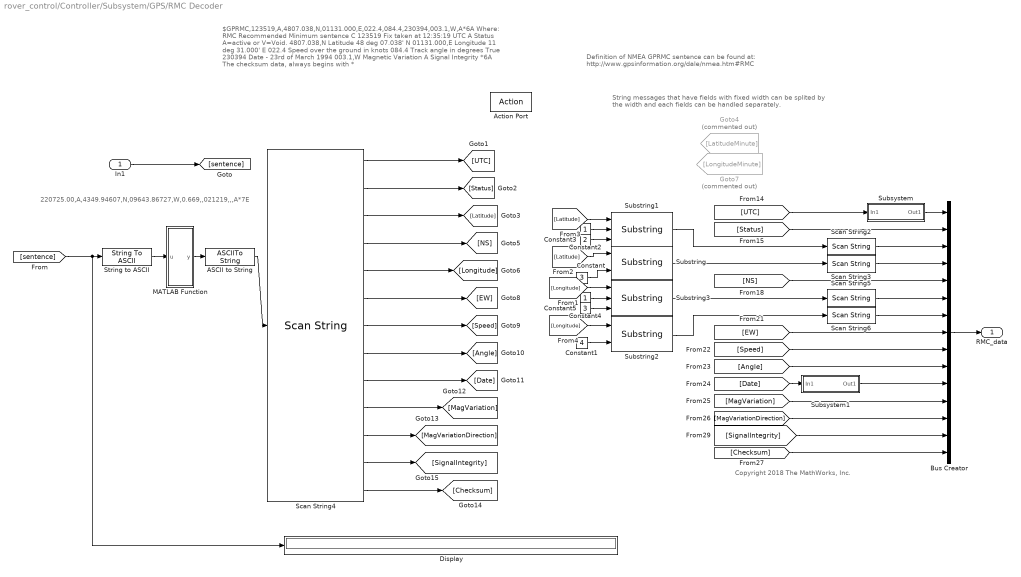
== system rover_control/Controller/Subsystem/GPS/RMC Decoder ==
  note: 220725.00,A,4349.94607,N,09643.86727,W,0.669,,021219,,,A*7E
  note: $GPRMC,123519,A,4807.038,N,01131.000,E,022.4,084.4,230394,003.1,W,A*6A
      | Where:
      | RMC          Recommended Minimum sentence C
      | 123519       Fix taken at 12:35:19 UTC
      | A            Status A=active or V=Void.
      | 4807.038,N   Latitude 48 deg 07.038' N
      | 01131.000,E  Longitude 11 deg 31.000' E
      | 022.4        Speed over the ground in knots
      | 084.4        Track angle in degrees True
      | 230394       Date - 23rd of March 1994
      | 003.1,W      Magnetic Variation
      | A			Signal Integrity
      | *6A          The checksum data, always begins with *
  note: Copyright 2018 The MathWorks, Inc.
  note: String messages that have fields with fixed width can be splited
      | by the width and each fields can be handled separately.
  note: Definition of NMEA GPRMC sentence can be found at:
      | http://www.gpsinformation.org/dale/nmea.htm#RMC
  In1 : Inport
  Action Port : ActionPort  ActionPortLabel=case [ RMC ]:
  ASCII to String : ASCIIToString
  Bus Creator : BusCreator  Inputs=15  OutDataTypeStr=Bus: NMEA_GPRMC  NonVirtualBus=on
      settings: InheritFromInputs=off
  Constant : Constant  Value=3  OutDataTypeStr=Inherit: Inherit via back propagation
  Constant1 : Constant  Value=4  OutDataTypeStr=Inherit: Inherit via back propagation
  Constant2 : Constant  OutDataTypeStr=Inherit: Inherit via back propagation
  Constant3 : Constant  Value=2  OutDataTypeStr=Inherit: Inherit via back propagation
  Constant4 : Constant  OutDataTypeStr=Inherit: Inherit via back propagation
  Constant5 : Constant  Value=3  OutDataTypeStr=Inherit: Inherit via back propagation
  Display : Display
  Goto4 : Goto  Commented=on  GotoTag=LatitudeMinute
  Goto7 : Goto  Commented=on  GotoTag=LongitudeMinute
  MATLAB Function : MATLAB Function  TreatAsAtomicUnit=on
  Scan String2 : ScanString  Format="\"%hu\""
  Scan String3 : ScanString  Format="\"%lf\""
  Scan String4 : ScanString  Format="\"%9s,%1s,%10s,%1s,%11s,%1s,%lf,%lf,%s,%lf,%s,%s,*%s\""
  Scan String5 : ScanString  Format="\"%hu\""
  Scan String6 : ScanString  Format="\"%lf\""
  String to ASCII : StringToASCII  OutputVectorSize=80
  Substring : Substring  StringFromIdxToEnd=on
  Substring1 : Substring
  Substring2 : Substring  StringFromIdxToEnd=on
  Substring3 : Substring
  Subsystem : Subsystem
  Subsystem1 : Subsystem
  RMC_data : Outport  VectorParamsAs1DForOutWhenUnconnected=off
  wires:
  In1/1 -> [sentence]
  Scan String4/1 -> [UTC]
  Scan String4/2 -> [Status]
  Scan String4/3 -> [Latitude]
  ? -> Goto4/1
  Scan String4/4 -> [NS]
  Scan String4/5 -> [Longitude]
  ? -> Goto7/1
  Scan String4/6 -> [EW]
  Scan String4/7 -> [Speed]
  Bus Creator/1 -> RMC_data/1
  [UTC] -> Subsystem/1(In1)
  [Status] -> Bus Creator/2
  [NS] -> Bus Creator/5
  [EW] -> Bus Creator/8
  [Date] -> Subsystem1/1(In1)
  [MagVariationDirection] -> Bus Creator/13
  [Checksum] -> Bus Creator/15
  Scan String3/1 -> Bus Creator/4
  Scan String5/1 -> Bus Creator/6
  Scan String6/1 -> Bus Creator/7
  [Speed] -> Bus Creator/9
  [Angle] -> Bus Creator/10
  [MagVariation] -> Bus Creator/12
  Subsystem/1(Out1) -> Bus Creator/1
  Subsystem1/1(Out1) -> Bus Creator/11
  [SignalIntegrity] -> Bus Creator/14
  [sentence] -> String to ASCII/1, Display/1
  Substring2/1 -> Scan String6/1
  Substring3/1 -> Scan String5/1
  Substring/1 -> Scan String3/1
  Constant2/1 -> Substring1/2
  Substring1/1 -> Scan String2/1
  [Longitude] -> Substring3/1
  [Latitude] -> Substring/1
  Constant5/1 -> Substring3/3
  [Latitude] -> Substring1/1
  Constant4/1 -> Substring3/2
  Constant1/1 -> Substring2/2
  Constant/1 -> Substring/2
  Constant3/1 -> Substring1/3
  [Longitude] -> Substring2/1
  Scan String2/1 -> Bus Creator/3
  String to ASCII/1 -> MATLAB Function/1(u)
  Scan String4/8 -> [Angle]
  Scan String4/10 -> [MagVariation]
  MATLAB Function/1(y) -> ASCII to String/1
  ASCII to String/1 -> Scan String4/1
  Scan String4/9 -> [Date]
  Scan String4/11 -> [MagVariationDirection]
  Scan String4/12 -> [SignalIntegrity]
  Scan String4/13 -> [Checksum]

== system rover_control/Controller/Subsystem/GPS/Unsupported ==
  In1 : Inport
  Action Port : ActionPort  ActionPortLabel=default:
  String Concatenate : StringConcatenate  Inputs=3
  String Constant : StringConstant  String="\"Message '\""
  String Constant1 : StringConstant  String="\"' is not supported!\""
  Out1 : Outport  VectorParamsAs1DForOutWhenUnconnected=off
  wires:
  In1/1 -> String Concatenate/2
  String Constant/1 -> String Concatenate/1
  String Constant1/1 -> String Concatenate/3
  String Concatenate/1 -> Out1/1

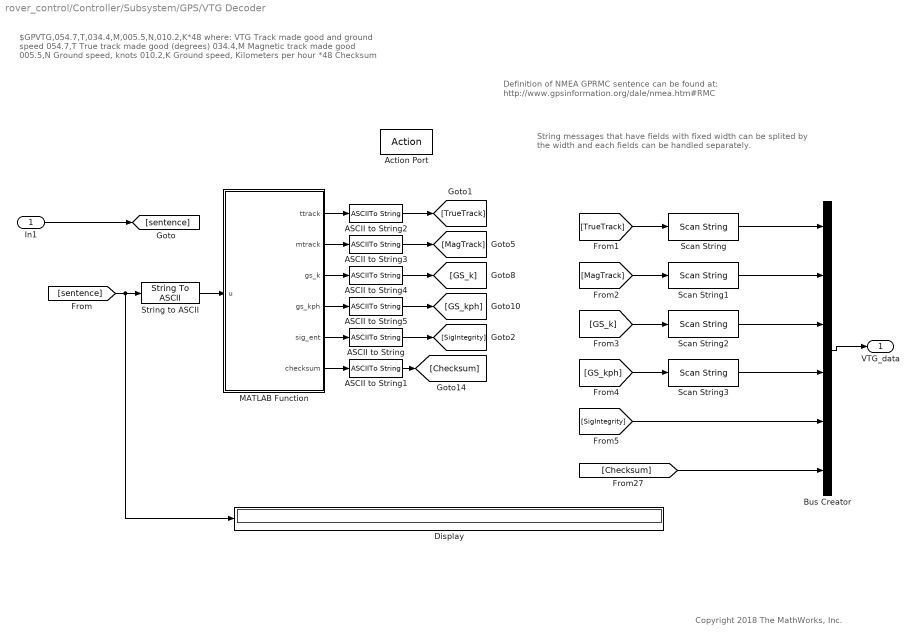
== system rover_control/Controller/Subsystem/GPS/VTG Decoder ==
  note: $GPVTG,054.7,T,034.4,M,005.5,N,010.2,K*48
      |
      | where:
      | VTG Track made good and ground speed
      | 054.7,T True track made good (degrees)
      | 034.4,M Magnetic track made good
      | 005.5,N Ground speed, knots
      | 010.2,K Ground speed, Kilometers per hour
      | *48 Checksum
  note: Copyright 2018 The MathWorks, Inc.
  note: String messages that have fields with fixed width can be splited
      | by the width and each fields can be handled separately.
  note: Definition of NMEA GPRMC sentence can be found at:
      | http://www.gpsinformation.org/dale/nmea.htm#RMC
  In1 : Inport
  Action Port : ActionPort  ActionPortLabel=case [ VTG ]:
  ASCII to String{,1..5} (6 alike) : ASCIIToString
  Bus Creator : BusCreator  Inputs=6  OutDataTypeStr=Bus: NMEA_VTG  NonVirtualBus=on
      settings: InheritFromInputs=off
  Display : Display
  MATLAB Function : MATLAB Function  TreatAsAtomicUnit=on
  Scan String{,1..3} (4 alike) : ScanString  Format="\"%lf\""
  String to ASCII : StringToASCII  OutputVectorSize=80
  VTG_data : Outport  VectorParamsAs1DForOutWhenUnconnected=off
  wires:
  In1/1 -> [sentence]
  Bus Creator/1 -> VTG_data/1
  [Checksum] -> Bus Creator/6
  [TrueTrack] -> Scan String/1
  [sentence] -> String to ASCII/1, Display/1
  MATLAB Function/6(checksum) -> ASCII to String1/1
  [MagTrack] -> Scan String1/1
  [GS_k] -> Scan String2/1
  [GS_kph] -> Scan String3/1
  MATLAB Function/5(sig_ent) -> ASCII to String/1
  [SigIntegrity] -> Bus Creator/5
  MATLAB Function/1(ttrack) -> ASCII to String2/1
  MATLAB Function/2(mtrack) -> ASCII to String3/1
  MATLAB Function/3(gs_k) -> ASCII to String4/1
  MATLAB Function/4(gs_kph) -> ASCII to String5/1
  String to ASCII/1 -> MATLAB Function/1(u)
  ASCII to String/1 -> [SigIntegrity]
  ASCII to String1/1 -> [Checksum]
  ASCII to String2/1 -> [TrueTrack]
  ASCII to String3/1 -> [MagTrack]
  ASCII to String4/1 -> [GS_k]
  ASCII to String5/1 -> [GS_kph]
  Scan String/1 -> Bus Creator/1
  Scan String1/1 -> Bus Creator/2
  Scan String2/1 -> Bus Creator/3
  Scan String3/1 -> Bus Creator/4

== system rover_control/Plant/Subsystem1/Subsystem1/MotorDrive ==
  dir : Inport
  en : Inport  Port=2  OutMin=0  OutMax=1
  Chart : Stateflow chart  BlockKeywords=__PRM__SERIALIZED__DATA__:Stateflow Chart,Stateflow Diagram  TreatAsAtomicUnit=on
  Enable : raspberrypilib/PWM  board=Pi 3 Model B+  Pin_=17  Frequency=4000  blockPlatform=Raspberry Pi
      settings: SourceProductName=Simulink Support Package for Raspberry Pi Hardware  SourceProductBaseCode=RASPPI
  Fwd : embdlinuxlib/GPIO Write  board=Pi 3 Model B+  gpio=27  direction=Output  blockPlatform=Raspberry Pi
      settings: SourceProductName=Simulink Support Package for Raspberry Pi Hardware  SourceProductBaseCode=RASPPI
  Rev : embdlinuxlib/GPIO Write  board=Pi 3 Model B+  gpio=18  direction=Output  blockPlatform=Raspberry Pi
      settings: SourceProductName=Simulink Support Package for Raspberry Pi Hardware  SourceProductBaseCode=RASPPI
  wires:
  dir/1 -> Chart/1(direction)
  en/1 -> Enable/1
  Chart/1(fwd) -> Fwd/1
  Chart/2(rev) -> Rev/1
